simulink model "VirtualDAQ"  (R2021b)
settings: Solver=VariableStepAuto  StartTime=0.0  StopTime=inf  MaxStep=0.001  RelTol=1e-3
libraries: fl_lib x5, simulink x3, nesl_utility x3, dspxfrm3 x1
(part 1 of 2)
settings Model: Creator=Work  LastModifiedBy=Work

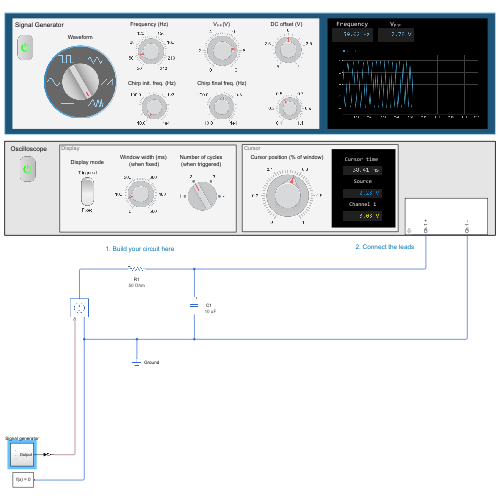
[thumbnail: Simulink's stored preview of the top-level diagram]
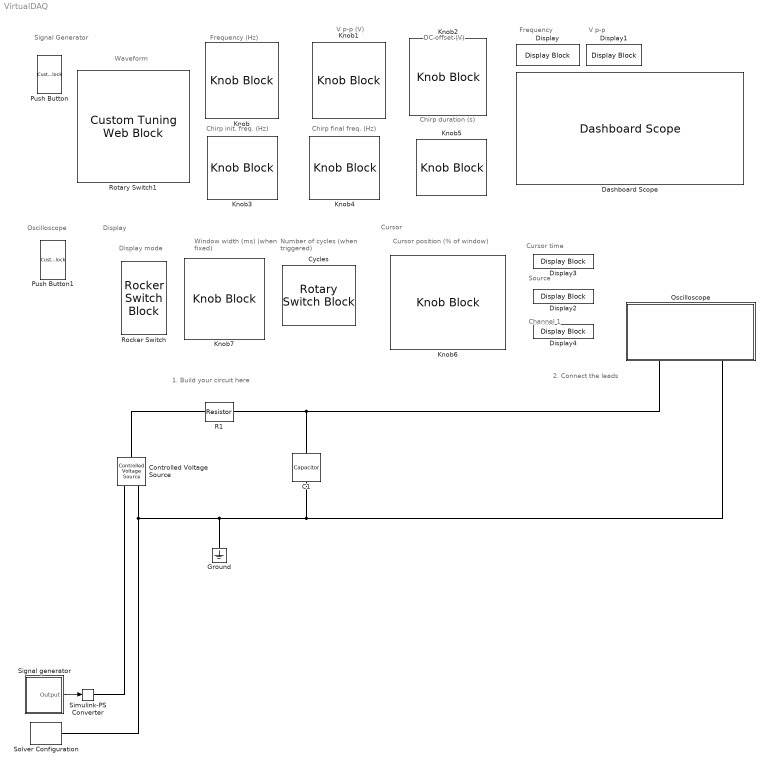
== system VirtualDAQ ==
  note: Display
  note: Cursor
  note: 1. Build your circuit here
  note: Frequency (Hz)
  note: Waveform
  note: V p-p (V)
  note: Signal Generator
  note: Oscilloscope
  note: Number of cycles
      | (when triggered)
  note: DC offset (V)
  note: Frequency
  note: V p-p
  note: Chirp init. freq. (Hz)
  note: Chirp final freq. (Hz)
  note: Chirp duration (s)
  note: Source
  note: 2. Connect the leads
  note: Cursor position (% of window)
  note: Channel 1
  note: Cursor time
  note: Display mode
  note: Window width (ms)
      | (when fixed)
  C1 : fl_lib/Electrical/Electrical Elements/Capacitor  c=10 uF  r=1e-6 Ohm  g=0 1/Ohm  i_specify=off  i_priority=None  i=0 A  i_nominal_specify=off  i_nominal_unit=A  i_nominal_value=1  v_specify=off  v_priority=None  v=0 V  v_nominal_specify=off  v_nominal_unit=V  v_nominal_value=1  vc_specify=off  vc_priority=High  vc=0 V  vc_nominal_specify=off  vc_nominal_unit=V  vc_nominal_value=1
      settings: AttributesFormatString=%<c> %<c_unit>
  Controlled Voltage Source : fl_lib/Electrical/Electrical Sources/Controlled Voltage Source
  Cycles : RotarySwitchBlock  LabelPosition=Hide
      settings: Values={{'1', '2', '3', '4'}, [1 2 3 4]}
  Dashboard Scope : DashboardScope  TimeSpan=0.20000000000000001  Ymin=-5  Ymax=5  ScaleAtStop=off
  Display : DisplayBlock  LabelPosition=Hide  Format=Custom  Alignment=Right  Transparency=1  FormatString=%0.2f Hz
  Display1 : DisplayBlock  LabelPosition=Hide  Format=Custom  Alignment=Right  Transparency=1  FormatString=%0.2f V
  Display2 : DisplayBlock  LabelPosition=Hide  Format=Custom  Alignment=Right  Transparency=1  FormatString=%0.2f V
  Display3 : DisplayBlock  LabelPosition=Hide  Format=Custom  Alignment=Right  Transparency=1  FormatString=%0.2f ms
  Display4 : DisplayBlock  LabelPosition=Hide  Format=Custom  Alignment=Right  Transparency=1  FormatString=%0.2f V
  Ground : fl_lib/Electrical/Electrical Elements/Electrical Reference
  Knob : KnobBlock  LabelPosition=Hide  ScaleMin=30  ScaleMax=240  TickInterval=30
  Knob1 : KnobBlock  LabelPosition=Hide  ScaleMax=10  TickInterval=2
  Knob2 : KnobBlock  LabelPosition=Hide  ScaleMin=-5  ScaleMax=5  TickInterval=2.5
  Knob3 : KnobBlock  LabelPosition=Hide  ScaleMin=10  ScaleMax=10000  ScaleType=Log
  Knob4 : KnobBlock  LabelPosition=Hide  ScaleMin=10  ScaleMax=10000  ScaleType=Log
  Knob5 : KnobBlock  LabelPosition=Hide  ScaleMin=0.1  ScaleMax=1.1  TickInterval=0.2
  Knob6 : KnobBlock  LabelPosition=Hide  ScaleMax=1  TickInterval=0.2
  Knob7 : KnobBlock  LabelPosition=Hide  ScaleMax=500  TickInterval=100
  Oscilloscope : Subsystem  mask{Np=256, plot_dt=0.5e-5, refreshRate=100}
      mask prompts: Np "Sample points"; plot_dt "Sample time (s)"; refreshRate "Plot refresh rate (Hz)"
      settings: PortSchema="{\"entries\":[{\"content\":{\"sides\":[{\"content\":{\"connectorIds\":[]},\"type\":\"ConnectorPlacement.EquallySpacedRectSide\",\"uuid\":\"cb438ba8-b2b3-45b1-8b71-f49eaacb653e\"},{\"content\":{\"connectorIds\":[],\"side\":\"RIGHT\"},\"type\":\"ConnectorPlacement.EquallySpacedRectSide\",\"uuid\":\"160127e0-8288-4de0-8c5e-c0f830785117\"},{\"content\":{\"connectorIds\":[],\"side\":\"TOP\"},\"type\":\"ConnectorPlacement.EquallySpacedRectSide\",\"uuid\":\"dfb316bc-2ce0-497e-8709-34b9c31010dc\"},{\"content\":{\"connectorIds\":[\"RConn1\",\"RConn2\"],\"side\":\"BOTTOM\"},\"type\":\"ConnectorPlacement.EquallySpacedRectSide\",\"uuid\":\"83fd5f15-dddb-40a3-a521-3544cb4554d5\"}]},\"type\":\"ConnectorPlacement.EquallySpacedConnector\",\"uuid\":\"afdb78c4-5eda-48fa-a0b8-f8a4ea028205\"}],\"packageUris\":[\"http://schema.mathworks.com/mf0/Connector/R2020b\"],\"version\":\"1.0\"}"
  Push Button : CustomTuningWebBlock  LabelPosition=Hide  ShowInitialText=on  Configuration="{\"components\":[{\"name\":\"BackgroundImageComponent\",\"settings\":{\"image\":{\"size\":[0,0],\"src\":\"default\",\"srcOrientation\":\"horizontal\"},\"position\":[0,0,1,1],\"scaleMode\":\"0\"}},{\"name\":\"ButtonStateComponent\",\"settings\":{\"buttonType\":\"latch\",\"clickFcn\":\"\",\"latched\":true,\"offValue\":0,\"onValue\":1,\"position\":[0,0,1,1],\"pressDelay\":500,\"pressFcn\":\"\",\"repeatInterval\":0,\"states\":[{\"horizontalAlignment\":\"center\",\"image\":{\"position\":[0,0.0025052342791134774,0.994989531441773,1],\"size\":[0.994989531441773,1],\"src\":\"data:image\\/png;base64,iVBORw0KGgoAAAANSUhEUgAAAUIAAAIBCAYAAAA8ibbDAAAACXBIWXMAAC4lAAAuJQH4pnvtAAAAGXRFWHRTb2Z0d2FyZQB3d3cuaW5rc2NhcGUub3Jnm+48GgAAIABJREFUeJzt3XeUZNd9H\\/jvfZW6q+N0dQ7TafIAkwAMhgAnSRZpWmFNUiBtWTbP+pBc7x9cmSbMJMzoEQ2IABcSRUmHe0RyvV6tJcuESItLShaDdHoG5BAYDIgwsSd1zjlUd3WFd\\/3HdDcmvFepq16o9\\/2cM4dEv\\/Tr6qpv3RfuvQJkuS9+8YsNHo+nTQjRBqBRCFENoBpAtRAiJKUMASgCUCSEKAYAKWUZAK9VNZOuuBBiEQCklCsAIkKIFSnltBBiWko5DWBK ...(+23218 chars)\",\"srcOrientation\":\"Right\"},\"label\":{\"color\":[0.9176470588235294,0.9176470588235294,0.9176470588235294],\"icon\":{\"size\":[0,0],\"src\":\"default\",\"srcOrientation\":\"Right\"},\"iconPlacement\":\"left\",\"opacity\":1,\"show\":true,\"text\":{\"content\":\"\",\"font\":\"Helvetica\",\"fontSize\":42}},\"labelOffset\":[-0.019507668917408183,0.0018518518518518268],\"verticalAlignment\":\"middle\"},{\"horizontalAlignment\":\"center\",\"image\":{\"position\":[0,0.0025052342791134774,0.994989531441773,1],\"size\":[0.994989531441773,1],\"src\":\"data:image\\/png;base64,iVBORw0KGgoAAAANSUhEUgAAAUIAAAIBCAYAAAA8ibbDAAAACXBIWXMAAC4lAAAuJQH4pnvtAAAAGXRFWHRTb2Z0d2FyZQB3d3cuaW5rc2NhcGUub3Jnm+48GgAAIABJREFUeJzs3Xd8HMd9N\\/7P7DXg0HFoBHsRxSKJIimJKiYJynGN4y7bcYqTPLZ\\/fl6\\/OLESxUUR6ZUgRcVyi\\/1zfrGdPC6xE1txkS07lixbBGV1yVRjETtBkACIeih3uLbz\\/IFCANzd293ba7jPOy85xO7M7PAIfDGz0wQo72699dZFHo9nhRBiBYBWIUQDgAYADUKIkJQyBKAMQJkQohwApJRVALz5qjPpSgohRgFAShkFMCGEiEopB4QQA1LKAQD9Usp+RV ...(+27278 chars)\",\"srcOrientation\":\"Right\"},\"label\":{\"color\":[0.9176470588235294,0.9176470588235294,0.9176470588235294],\"icon\":{\"size\":[0,0],\"src\":\"default\",\"srcOrientation\":\"Right\"},\"iconPlacement\":\"top\",\"opacity\":1,\"show\":true,\"text\":{\"content\":\"\",\"font\":\"Helvetica\",\"fontSize\":42}},\"labelOffset\":[-0.017384370015948947,0.002777777777777768],\"verticalAlignment\":\"middle\"},{\"horizontalAlignment\":\"center\",\"image\":{\"position\":[0,0.0025052342791134774,0.994989531441773,1],\"size\":[0.994989531441773,1],\"src\":\"data:image\\/png;base64,iVBORw0KGgoAAAANSUhEUgAAAUIAAAIBCAYAAAA8ibbDAAAACXBIWXMAAC4lAAAuJQH4pnvtAAAAGXRFWHRTb2Z0d2FyZQB3d3cuaW5rc2NhcGUub3Jnm+48GgAAIABJREFUeJzs3Xd8HMd9N\\/7P7DXg0HFoBHsRxSKJIimJKiYJynGN4y7bcYqTPLZ\\/fl6\\/OLESxUUR6ZUgRcVyi\\/1zfrGdPC6xE1txkS07lixbBGV1yVRjETtBkACIeih3uLbz\\/IFCANzd293ba7jPOy85xO7M7PAIfDGz0wQo72699dZFHo9nhRBiBYBWIUQDgAYADUKIkJQyBKAMQJkQohwApJRVALz5qjPpSgohRgFAShkFMCGEiEopB4QQA1LKAQD9Usp+RV ...(+27278 chars)\",\"srcOrientation\":\"Right\"},\"label\":{\"color\":[0.9176470588235294,0.9176470588235294,0.9176470588235294],\"icon\":{\"size\":[0,0],\"src\":\"default\",\"srcOrientation\":\"Right\"},\"iconPlacement\":\"left\",\"opacity\":1,\"show\":true,\"text\":{\"content\":\"\",\"font\":\"Helvetica\",\"fontSize\":21}},\"labelOffset\":[0,0],\"verticalAlignment\":\"middle\"},{\"horizontalAlignment\":\"center\",\"image\":{\"position\":[0,0.0025052342791134774,0.994989531441773,1],\"size\":[0.994989531441773,1],\"src\":\"data:image\\/png;base64,iVBORw0KGgoAAAANSUhEUgAAAUIAAAIBCAYAAAA8ibbDAAAACXBIWXMAAC4lAAAuJQH4pnvtAAAAGXRFWHRTb2Z0d2FyZQB3d3cuaW5rc2NhcGUub3Jnm+48GgAAIABJREFUeJzs3Xd8HMd9N\\/7P7DXg0HFoBHsRxSKJIimJKiYJynGN4y7bcYqTPLZ\\/fl6\\/OLESxUUR6ZUgRcVyi\\/1zfrGdPC6xE1txkS07lixbBGV1yVRjETtBkACIeih3uLbz\\/IFCANzd293ba7jPOy85xO7M7PAIfDGz0wQo72699dZFHo9nhRBiBYBWIUQDgAYADUKIkJQyBKAMQJkQohwApJRVALz5qjPpSgohRgFAShkFMCGEiEopB4QQA1LKAQD9Usp+RV ...(+27278 chars)\",\"srcOrientation\":\"Right\"},\"label\":{\"color\":[0.9176470588235294,0.9176470588235294,0.9176470588235294],\"icon\":{\"size\":[0,0],\"src\":\"default\",\"srcOrientation\":\"Right\"},\"iconPlacement\":\"left\",\"opacity\":1,\"show\":true,\"text\":{\"content\":\"\",\"font\":\"Helvetica\",\"fontSize\":21}},\"labelOffset\":[0.025,0],\"verticalAlignment\":\"middle\"}]}},{\"name\":\"ForegroundImageComponent\",\"settings\":{\"image\":{\"size\":[0,0],\"src\":\"default\",\"srcOrientation\":\"horizontal\"},\"isForeground\":1,\"position\":[0,0,1,1],\"scaleMode\":\"0\"}}],\"settings\":{\"BindingType\":\"param\",\"aspectRatio\":3.7777777777777777,\"backgroundColor\":[0,0,0,\"1\"],\"backgroundOffset\":0,\"backgroundOpacity\":1,\"fixedAspectRatio\":\"on\",\"foregroundColor\":[252,252,196],\"showBackgroundColor\":false,\"variant\":\"push\"},\"type\":\"Button\"}"
  Push Button1 : CustomTuningWebBlock  LabelPosition=Hide  ShowInitialText=on  Configuration="{\"components\":[{\"name\":\"BackgroundImageComponent\",\"settings\":{\"image\":{\"size\":[0,0],\"src\":\"default\",\"srcOrientation\":\"horizontal\"},\"position\":[0,0,1,1],\"scaleMode\":\"0\"}},{\"name\":\"ButtonStateComponent\",\"settings\":{\"buttonType\":\"latch\",\"clickFcn\":\"\",\"latched\":true,\"offValue\":0,\"onValue\":1,\"position\":[0,0,1,1],\"pressDelay\":500,\"pressFcn\":\"\",\"repeatInterval\":0,\"states\":[{\"horizontalAlignment\":\"center\",\"image\":{\"position\":[0,0.0025052342791134774,0.994989531441773,1],\"size\":[0.994989531441773,1],\"src\":\"data:image\\/png;base64,iVBORw0KGgoAAAANSUhEUgAAAUIAAAIBCAYAAAA8ibbDAAAACXBIWXMAAC4lAAAuJQH4pnvtAAAAGXRFWHRTb2Z0d2FyZQB3d3cuaW5rc2NhcGUub3Jnm+48GgAAIABJREFUeJzt3XeUZNd9H\\/jvfZW6q+N0dQ7TafIAkwAMhgAnSRZpWmFNUiBtWTbP+pBc7x9cmSbMJMzoEQ2IABcSRUmHe0RyvV6tJcuESItLShaDdHoG5BAYDIgwsSd1zjlUd3WFd\\/3HdDcmvFepq16o9\\/2cM4dEv\\/Tr6qpv3RfuvQJkuS9+8YsNHo+nTQjRBqBRCFENoBpAtRAiJKUMASgCUCSEKAYAKWUZAK9VNZOuuBBiEQCklCsAIkKIFSnltBBiWko5DWBK ...(+23218 chars)\",\"srcOrientation\":\"Right\"},\"label\":{\"color\":[0.9176470588235294,0.9176470588235294,0.9176470588235294],\"icon\":{\"size\":[0,0],\"src\":\"default\",\"srcOrientation\":\"Right\"},\"iconPlacement\":\"left\",\"opacity\":1,\"show\":true,\"text\":{\"content\":\"\",\"font\":\"Helvetica\",\"fontSize\":42}},\"labelOffset\":[-0.019507668917408183,0.0018518518518518268],\"verticalAlignment\":\"middle\"},{\"horizontalAlignment\":\"center\",\"image\":{\"position\":[0,0.0025052342791134774,0.994989531441773,1],\"size\":[0.994989531441773,1],\"src\":\"data:image\\/png;base64,iVBORw0KGgoAAAANSUhEUgAAAUIAAAIBCAYAAAA8ibbDAAAACXBIWXMAAC4lAAAuJQH4pnvtAAAAGXRFWHRTb2Z0d2FyZQB3d3cuaW5rc2NhcGUub3Jnm+48GgAAIABJREFUeJzs3Xd8HMd9N\\/7P7DXg0HFoBHsRxSKJIimJKiYJynGN4y7bcYqTPLZ\\/fl6\\/OLESxUUR6ZUgRcVyi\\/1zfrGdPC6xE1txkS07lixbBGV1yVRjETtBkACIeih3uLbz\\/IFCANzd293ba7jPOy85xO7M7PAIfDGz0wQo72699dZFHo9nhRBiBYBWIUQDgAYADUKIkJQyBKAMQJkQohwApJRVALz5qjPpSgohRgFAShkFMCGEiEopB4QQA1LKAQD9Usp+RV ...(+27278 chars)\",\"srcOrientation\":\"Right\"},\"label\":{\"color\":[0.9176470588235294,0.9176470588235294,0.9176470588235294],\"icon\":{\"size\":[0,0],\"src\":\"default\",\"srcOrientation\":\"Right\"},\"iconPlacement\":\"top\",\"opacity\":1,\"show\":true,\"text\":{\"content\":\"\",\"font\":\"Helvetica\",\"fontSize\":42}},\"labelOffset\":[-0.017384370015948947,0.002777777777777768],\"verticalAlignment\":\"middle\"},{\"horizontalAlignment\":\"center\",\"image\":{\"position\":[0,0.0025052342791134774,0.994989531441773,1],\"size\":[0.994989531441773,1],\"src\":\"data:image\\/png;base64,iVBORw0KGgoAAAANSUhEUgAAAUIAAAIBCAYAAAA8ibbDAAAACXBIWXMAAC4lAAAuJQH4pnvtAAAAGXRFWHRTb2Z0d2FyZQB3d3cuaW5rc2NhcGUub3Jnm+48GgAAIABJREFUeJzs3Xd8HMd9N\\/7P7DXg0HFoBHsRxSKJIimJKiYJynGN4y7bcYqTPLZ\\/fl6\\/OLESxUUR6ZUgRcVyi\\/1zfrGdPC6xE1txkS07lixbBGV1yVRjETtBkACIeih3uLbz\\/IFCANzd293ba7jPOy85xO7M7PAIfDGz0wQo72699dZFHo9nhRBiBYBWIUQDgAYADUKIkJQyBKAMQJkQohwApJRVALz5qjPpSgohRgFAShkFMCGEiEopB4QQA1LKAQD9Usp+RV ...(+27278 chars)\",\"srcOrientation\":\"Right\"},\"label\":{\"color\":[0.9176470588235294,0.9176470588235294,0.9176470588235294],\"icon\":{\"size\":[0,0],\"src\":\"default\",\"srcOrientation\":\"Right\"},\"iconPlacement\":\"left\",\"opacity\":1,\"show\":true,\"text\":{\"content\":\"\",\"font\":\"Helvetica\",\"fontSize\":21}},\"labelOffset\":[0,0],\"verticalAlignment\":\"middle\"},{\"horizontalAlignment\":\"center\",\"image\":{\"position\":[0,0.0025052342791134774,0.994989531441773,1],\"size\":[0.994989531441773,1],\"src\":\"data:image\\/png;base64,iVBORw0KGgoAAAANSUhEUgAAAUIAAAIBCAYAAAA8ibbDAAAACXBIWXMAAC4lAAAuJQH4pnvtAAAAGXRFWHRTb2Z0d2FyZQB3d3cuaW5rc2NhcGUub3Jnm+48GgAAIABJREFUeJzs3Xd8HMd9N\\/7P7DXg0HFoBHsRxSKJIimJKiYJynGN4y7bcYqTPLZ\\/fl6\\/OLESxUUR6ZUgRcVyi\\/1zfrGdPC6xE1txkS07lixbBGV1yVRjETtBkACIeih3uLbz\\/IFCANzd293ba7jPOy85xO7M7PAIfDGz0wQo72699dZFHo9nhRBiBYBWIUQDgAYADUKIkJQyBKAMQJkQohwApJRVALz5qjPpSgohRgFAShkFMCGEiEopB4QQA1LKAQD9Usp+RV ...(+27278 chars)\",\"srcOrientation\":\"Right\"},\"label\":{\"color\":[0.9176470588235294,0.9176470588235294,0.9176470588235294],\"icon\":{\"size\":[0,0],\"src\":\"default\",\"srcOrientation\":\"Right\"},\"iconPlacement\":\"left\",\"opacity\":1,\"show\":true,\"text\":{\"content\":\"\",\"font\":\"Helvetica\",\"fontSize\":21}},\"labelOffset\":[0.025,0],\"verticalAlignment\":\"middle\"}]}},{\"name\":\"ForegroundImageComponent\",\"settings\":{\"image\":{\"size\":[0,0],\"src\":\"default\",\"srcOrientation\":\"horizontal\"},\"isForeground\":1,\"position\":[0,0,1,1],\"scaleMode\":\"0\"}}],\"settings\":{\"BindingType\":\"param\",\"aspectRatio\":3.7777777777777777,\"backgroundColor\":[0,0,0,\"1\"],\"backgroundOffset\":0,\"backgroundOpacity\":1,\"fixedAspectRatio\":\"on\",\"foregroundColor\":[252,252,196],\"showBackgroundColor\":false,\"variant\":\"push\"},\"type\":\"Button\"}"
  R1 : fl_lib/Electrical/Electrical Elements/Resistor  R=50 Ohm  i_specify=off  i_priority=None  i=0 A  i_nominal_specify=off  i_nominal_unit=A  i_nominal_value=1  v_specify=off  v_priority=None  v=0 V  v_nominal_specify=off  v_nominal_unit=V  v_nominal_value=1
      settings: AttributesFormatString=%<R> %<R_unit>
  Rocker Switch : RockerSwitchBlock  LabelPosition=Hide
      settings: Values={{'Fixed', 'Triggered'}, [0 1]}
  Rotary Switch1 : CustomTuningWebBlock  LabelPosition=Hide  ShowInitialText=on  Configuration="{\"components\":[{\"name\":\"RotarySwitchComponent\",\"settings\":{\"arcAngle\":300,\"arcAngleOffset\":120,\"handle\":{\"size\":[150,150],\"src\":\"data:image\\/svg+xml;base64,PHN2ZyBpZD0iTGF5ZXJfMSIgZGF0YS1uYW1lPSJMYXllciAxIiB4bWxucz0iaHR0cDovL3d3dy53My5vcmcvMjAwMC9zdmciIHhtbG5zOnhsaW5rPSJodHRwOi8vd3d3LnczLm9yZy8xOTk5L3hsaW5rIiB2aWV3Qm94PSIwIDAgMTIxIDEyMSI+PGRlZnM+PHN0eWxlPi5jbHMtMXtmaWxsOnVybCgjbGluZWFyLWdyYWRpZW50KTt9LmNscy0yLC5jbHMtM3tmaWxsOiNkMWQxZDE7fS5jbHMtM3tzdHJva2U6I2I3YjdiNztzdHJva2UtbWl0ZXJsaW1pdDoxMDtzdHJva2Utd2lkdGg6MC4yNXB4O30uY2xzLTR7ZmlsbDojZjMwMDAwO30uY2xzLTV7ZmlsbDojZjIxNzY3O308L3N0eWxlPjxsaW5lYXJHcmFkaWVudCBpZD0ibGluZWFyLWdyYWRpZW50IiB4MT0iNjAuNSIgeTE9IjEyMC41IiB4Mj0iNjAuNSIgeTI9IjAuNSIgZ3JhZGllbnRVbml0cz0idXNlclNwYWNlT25Vc2UiPjxzdG9wIG9mZnNldD0iMCIgc3RvcC1jb2xvcj0iI2QxZDFkMSIvPjxzdG9wIG9mZnNldD0iMC4xIiBzdG9wLWNvbG9yPSIjY2VjZWNlIi8+PHN0b3Agb2Zmc2V0PSIwLjE5IiBzdG9wLWNvbG9yPSIjYzNjM2MzIi8+PHN0b3Agb2Zmc2V0PSIwLjI4IiBzdG9wLWNvbG9yPSIjYjFiMWIxIi8+PHN0b3Agb2Zmc2V0PSIwLjM2IiBzdG9wLWNvbG9yPSIjOTg5ODk4Ii8+PHN0b3Agb2Zmc2V0PSIwLjQ0IiBzdG9wLWNvbG9yPSIjNzg3ODc4Ii8+PHN0b3Agb2Zmc2V0PSIwLjQ2IiBzdG9wLWNvbG9yPSIjNmI2YjZiIi8+PHN0b3Agb2Zmc2V0PSIwLjU0IiBzdG9wLWNvbG9yPSIjNmI2YjZiIi8+PHN0b3Agb2Zmc2V0PSIwLjU2IiBzdG9wLWNvbG9yPSIjNzY3Njc2Ii8+PHN0b3Agb2Zmc2V0PSIwLjY0IiBzdG9wLWNvbG9yPSIjOTc5Nzk3Ii8+PHN0b3Agb2Zmc2V0PSIwLjcyIiBzdG9wLWNvbG9yPSIjYjBiMGIwIi8+PHN0b3Agb2Zmc2V0PSIwLjgxIiBzdG9wLWNvbG9yPSIjYzNjM2MzIi8+PHN0b3Agb2Zmc2V0PSIwLjkiIHN0b3AtY29sb3I9IiNjZGNkY2QiLz48c3RvcCBvZmZzZXQ9IjEiIHN0b3AtY29sb3I9IiNkMWQxZDEiLz48L2xpbmVhckdyYWRpZW50PjwvZGVmcz48Y2lyY2xlIGNsYXNzPSJjbHMtMSIgY3g9IjYwLjUiIGN5PSI2MC41IiByPSI2MCIvPjxwYXRoIGNsYXNzPSJjbHMtMiIgZD0iTTYwLjUsMUE1OS41LDU5LjUsMCwxLDEsMSw2MC41LDU5LjU3LDU5LjU3LDAsMCwxLDYwLjUsMW0wLTFBNjAuNSw2MC41LDAsMSwwLDEyMSw2MC41LDYwLjUsNjAuNSwwLDAsMCw2MC41LDBaIi8+PHJlY3QgY2xhc3M9ImNscy0zIiB4PSIwLjUiIHk9IjUxLjUiIHdpZHRoPSIxMjAiIGhlaWdodD0iMTgiIHJ4PSIzLjA0Ii8+PHJlY3QgY2xhc3M9ImNscy00IiB4PSI1Ljc1IiB5PSI1OC43NSIgd2lkdGg9IjE2IiBoZWlnaHQ9IjMiLz48cGF0aCBjbGFzcz0iY2xzLTUiIGQ9Ik0yMS4yNSw1OS4yNXYyaC0xNXYtMmgxNW0xLTFoLTE3djRoMTd2LTRaIi8+PC9zdmc+\"},\"handleOffset\":[0,0],\"handleOrientation\":180,\"handlePosition\":[0,0,1,1],\"handleSize\":{\"height\":0.5,\"width\":0.5},\"labelRadius\":0.36,\"position\":[0,0,1,1],\"states\":[{\"Label\":{\"color\":[0,0,0,1],\"icon\":{\"size\":[0,0],\"src\":[],\"srcOrientation\":\"Right\"},\"iconPlacement\":\"left\",\"opacity\":1,\"position\":[0.7345552884615385,0.6796274038461538],\"show\":true,\"text\":{\"content\":\"0\",\"font\":\"Helvetica\",\"fontSize\":24}},\"Value\":0},{\"Label\":{\"color\":[0,0,0,1],\"icon\":{\"size\":[0,0],\"src\":[],\"srcOrientation\":\"Right\"},\"iconPlacement\":\"left\",\"opacity\":1,\"position\":[0.35757211538461536,0.7603966346153846],\"show\":true,\"text\":{\"content\":\"1\",\"font\":\"Helvetica\",\"fontSize\":24}},\"Value\":1},{\"Label\":{\"color\":[0,0,0,1],\"icon\":{\"size\":[0,0],\"src\":[],\"srcOrientation\":\"Right\"},\"iconPlacement\":\"left\",\"opacity\":1,\"position\":[0.09603365384615385,0.46033653846153844],\"show\":true,\"text\":{\"content\":\"2\",\"font\":\"Helvetica\",\"fontSize\":24}},\"Value\":2},{\"Label\":{\"color\":[0,0,0,1],\"icon\":{\"size\":[0,0],\"src\":[],\"srcOrientation\":\"Right\"},\"iconPlacement\":\"left\",\"opacity\":1,\"position\":[0.36532451923076925,0.1180889423076923],\"show\":true,\"text\":{\"content\":\"3\",\"font\":\"Helvetica\",\"fontSize\":24}},\"Value\":3},{\"Label\":{\"color\":[0,0,0,1],\"icon\":{\"size\":[0,0],\"src\":[],\"srcOrientation\":\"Right\"},\"iconPlacement\":\"left\",\"opacity\":1,\"position\":[0.7191706730769231,0.19501201923076922],\"show\":true,\"text\":{\"content\":\"4\",\"font\":\"Helvetica\",\"fontSize\":24}},\"Value\":4},{\"Label\":{\"color\":[0,0,0],\"icon\":{\"size\":[1,1],\"src\":\"default\",\"srcOrientation\":\"Right\"},\"iconPlacement\":\"left\",\"opacity\":1,\"position\":[0,0],\"show\":true,\"text\":{\"content\":\"5\",\"fontSize\":14}},\"Value\":5}],\"tickRadius\":0.32}},{\"name\":\"BackgroundImageComponent\",\"settings\":{\"image\":{\"size\":[691,691],\"src\":\"data:image\\/png;base64,iVBORw0KGgoAAAANSUhEUgAAArMAAAKzCAYAAAAN54UbAAAACXBIWXMAAB7lAAAe5QGuvPLVAAAAGXRFWHRTb2Z0d2FyZQB3d3cuaW5rc2NhcGUub3Jnm+48GgAAIABJREFUeJzs3XlgVNX9NvDn3Fky2feFhAQSAkSCoLjigqAoCuJSFde27ra2te2vrVrtki7Wttra5a3VuuC+oLiiiCIBwg6CLGEPWYEsZN+TmXveP0IwQGaSzD2T2Z7PH5q5Z+6534Ew8+Tm3u8RICIKQjcsWBPqqLfGWDQRo2siRgIxUiBGA2IkRAyEjNagxQjALCGiIKRNQIQCMkIAFgkZIyAEgHAIWAFAfDO9GUDkscdC9I41A7Af91yBLgCtApAAGgTQLQVahESbEOiE ...(+67388 chars)\",\"srcOrientation\":\"Right\"},\"position\":[0,0,1,1],\"scaleMode\":\"0\"}},{\"name\":\"ForegroundImageComponent\",\"settings\":{\"image\":{\"size\":[0,0],\"src\":\"default\",\"srcOrientation\":[]},\"isForeground\":1,\"position\":[0,0,1,1],\"scaleMode\":\"0\"}}],\"settings\":{\"BindingType\":\"param\",\"backgroundColor\":[0,0,255,\"1\"],\"enumDataType\":\"\",\"fixedAspectRatio\":\"on\",\"image\":{\"size\":[150,150],\"src\":\"data:image\\/svg+xml;base64,PD94bWwgdmVyc2lvbj0iMS4wIiBlbmNvZGluZz0iVVRGLTgiIHN0YW5kYWxvbmU9Im5vIj8+CjwhLS0gR2VuZXJhdG9yOiBBZG9iZSBJbGx1c3RyYXRvciAxOS4yLjEsIFNWRyBFeHBvcnQgUGx1Zy1JbiAuIFNWRyBWZXJzaW9uOiA2LjAwIEJ1aWxkIDApICAtLT4KCjxzdmcKICAgeG1sbnM6ZGM9Imh0dHA6Ly9wdXJsLm9yZy9kYy9lbGVtZW50cy8xLjEvIgogICB4bWxuczpjYz0iaHR0cDovL2NyZWF0aXZlY29tbW9ucy5vcmcvbnMjIgogICB4bWxuczpyZGY9Imh0dHA6Ly93d3cudzMub3JnLzE5OTkvMDIvMjItcmRmLXN5bnRh ...(+9660 chars)\"},\"showBackgroundColor\":false,\"useEnumDataType\":false,\"variant\":\"rotarySwitch\"},\"type\":\"RotarySwitch\"}"
  Signal generator : Subsystem
  Simulink-PS Converter : nesl_utility/Simulink-PS Converter  PhysicalDomain=network_engine_domain  SubClassName=ps_input  LeftPortType=input  RightPortType=output  PseudoPeriodic=off  Frequencies=[]  NoiseDistribution=none  NoiseParameters=[]  Unit=1  AffineConversion=off  FilteringAndDerivatives=provide  SimscapeFilterOrder=1  InputFilterTimeConstant=0.001  UdotUserProvided=0
      settings: SourceProductBaseCode=PW,SS
  Solver Configuration : nesl_utility/Solver Configuration  PhysicalDomain=network_engine_domain  SubClassName=solver  LeftPortType=input  RightPortType=generic  Tones=[]  Harmonics=[]  SimulateNoise=off  Profile=off  UseLocalSampling=off  EnableSwitchedLinearOptims=on  FrequencyDomain=off  UseCCode=off  RelTol=0.001  AbsTol=1e-06  MinStep=1e-09  ToWorkspace=off  RevertToSquareIcSolve=off  NumHomotopyIterations=100  PhasorMode=off  PhasorModeNumHarmonics=1  DoDC=off  ResidualTolerance=1e-09  UseLocalSolver=off  LocalSolverChoice=NE_BACKWARD_EULER_ADVANCER  LocalSolverSampleTime=0.001  DoFixedCost=off  MaxNonlinIter=3  MaxModeIter=2  ComputeImpulses=off  ImpulseIterations=2  LinearAlgebra=auto  EquationFormulation=NE_TIME_EF  DelaysMemoryBudget=1024  AutomaticFiltering=on  FilteringTimeConstant=0.001  PartitionStorageMethod=AS_NEEDED  PartitionMemoryBudget=1024  PartitionMethod=ROBUST
      settings: SourceProductBaseCode=PW,SS
  wires:
  Signal generator/1(Output) -> Simulink-PS Converter/1
  connections:
  Controlled Voltage Source/RConn2 -- Solver Configuration/RConn1 -- Ground/LConn1 -- C1/RConn1 -- Oscilloscope/RConn2
  C1/LConn1 -- Oscilloscope/RConn1 -- R1/RConn1
  Controlled Voltage Source/LConn1 -- R1/LConn1
  Simulink-PS Converter/RConn1 -- Controlled Voltage Source/RConn1
